simulink model "linkjifen"  (R2023a)
settings: Solver=VariableStepAuto  StartTime=0.0  StopTime=100  RelTol=1e-3
undefined symbols (not defined in the file or in its folder): sque
settings Model: Creator=Lenovo  LastModifiedBy=17634948724

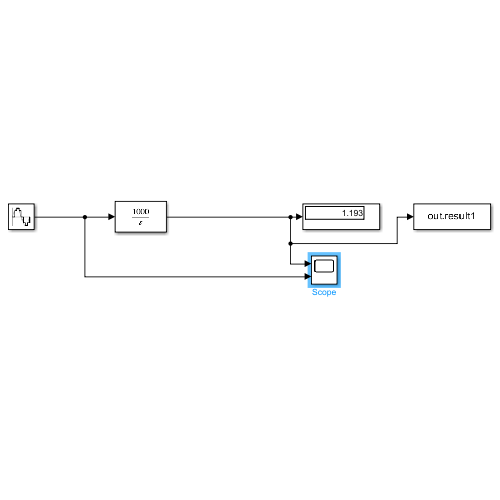
[thumbnail: Simulink's stored preview of the top-level diagram]
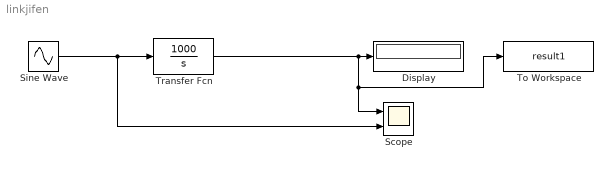
== system linkjifen ==
  Display : Display
  Scope : Scope  NumInputPorts=2
  Sine Wave : Sin  Amplitude=0.1  Frequency=sque  SampleTime=0.1
  To Workspace : ToWorkspace  VariableName=result1  SaveFormat=Timeseries  SampleTime=-1
  Transfer Fcn : TransferFcn  Numerator=[1000]  Denominator=[1 0]
  wires:
  Sine Wave/1 -> Transfer Fcn/1, Scope/2
  Transfer Fcn/1 -> To Workspace/1, Scope/1, Display/1
